simulink model "controller_test_2006"  (Simulink 6.4)
settings: Solver=ode45  StartTime=0.0  StopTime=10.0  RelTol=1e-3
values from neighbouring files (symbols this model uses):
  fundamental_sample_time = 0.01    [param_list.m]
  motor_stopped_value = DA_max / 2    [param_list.m]
libraries: simulink x1
settings Model: LastModifiedBy=Developer

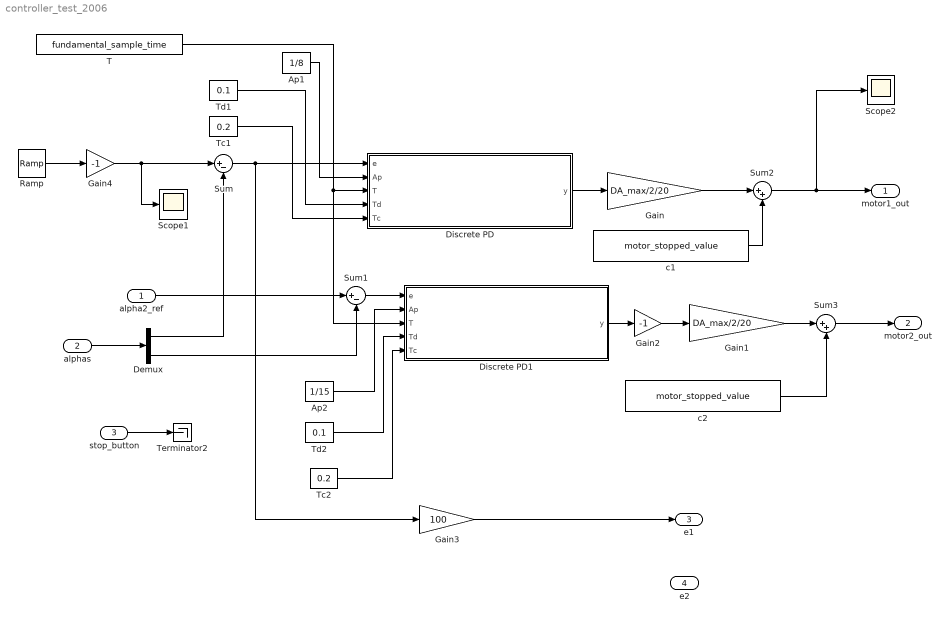
== system controller_test_2006 ==
  alpha2_ref : Inport
  alphas : Inport  Port=2
  stop_button : Inport  Port=3
  Ap1 : Constant  Value=1/8  OutDataType=sfix(16)  ConRadixGroup=Use specified scaling  OutScaling=2^0  SampleTime=inf  FramePeriod=inf
  Ap2 : Constant  Value=1/15  OutDataType=sfix(16)  ConRadixGroup=Use specified scaling  OutScaling=2^0  SampleTime=inf  FramePeriod=inf
  Demux : Demux  Outputs=2
  Discrete PD : Subsystem
  Discrete PD1 : Subsystem
  Gain : Gain  Gain=DA_max/2/20
  Gain1 : Gain  Gain=DA_max/2/20
  Gain2 : Gain  Gain=-1
  Gain3 : Gain  Gain=100
  Gain4 : Gain  Gain=-1
  Ramp : simulink/Sources/Ramp  SystemSampleTime=-1  slope=1  start=0  X0=0
  Scope1 : Scope
  Scope2 : Scope
  Sum : Sum  Inputs=|+-
  Sum1 : Sum  Inputs=|+-
  Sum2 : Sum  Inputs=|++
  Sum3 : Sum  Inputs=|++
  T : Constant  Value=fundamental_sample_time  OutDataType=sfix(16)  ConRadixGroup=Use specified scaling  OutScaling=2^0  SampleTime=inf  FramePeriod=inf
  Tc1 : Constant  Value=0.2  OutDataType=sfix(16)  ConRadixGroup=Use specified scaling  OutScaling=2^0  SampleTime=inf  FramePeriod=inf
  Tc2 : Constant  Value=0.2  OutDataType=sfix(16)  ConRadixGroup=Use specified scaling  OutScaling=2^0  SampleTime=inf  FramePeriod=inf
  Td1 : Constant  Value=0.1  OutDataType=sfix(16)  ConRadixGroup=Use specified scaling  OutScaling=2^0  SampleTime=inf  FramePeriod=inf
  Td2 : Constant  Value=0.1  OutDataType=sfix(16)  ConRadixGroup=Use specified scaling  OutScaling=2^0  SampleTime=inf  FramePeriod=inf
  Terminator2 : Terminator
  c1 : Constant  Value=motor_stopped_value  OutDataType=sfix(16)  ConRadixGroup=Use specified scaling  OutScaling=2^0  SampleTime=inf  FramePeriod=inf
  c2 : Constant  Value=motor_stopped_value  OutDataType=sfix(16)  ConRadixGroup=Use specified scaling  OutScaling=2^0  SampleTime=inf  FramePeriod=inf
  motor1_out : Outport
  motor2_out : Outport  Port=2
  e1 : Outport  Port=3
  e2 : Outport  Port=4
  wires:
  stop_button/1 -> Terminator2/1
  alphas/1 -> Demux/1
  Ramp/1 -> Gain4/1
  Sum/1 -> Discrete PD/1(e), Gain3/1
  Ap1/1 -> Discrete PD/2(Ap)
  T/1 -> Discrete PD/3(T), Discrete PD1/3(T)
  Td1/1 -> Discrete PD/4(Td)
  Tc1/1 -> Discrete PD/5(Tc)
  Demux/1 -> Sum/2
  Sum1/1 -> Discrete PD1/1(e)
  alpha2_ref/1 -> Sum1/1
  Demux/2 -> Sum1/2
  Ap2/1 -> Discrete PD1/2(Ap)
  Td2/1 -> Discrete PD1/4(Td)
  Tc2/1 -> Discrete PD1/5(Tc)
  Discrete PD1/1(y) -> Gain2/1
  Gain2/1 -> Gain1/1
  Gain3/1 -> e1/1
  Discrete PD/1(y) -> Gain/1
  c1/1 -> Sum2/2
  Gain/1 -> Sum2/1
  Sum2/1 -> motor1_out/1, Scope2/1
  Gain4/1 -> Sum/1, Scope1/1
  c2/1 -> Sum3/2
  Gain1/1 -> Sum3/1
  Sum3/1 -> motor2_out/1

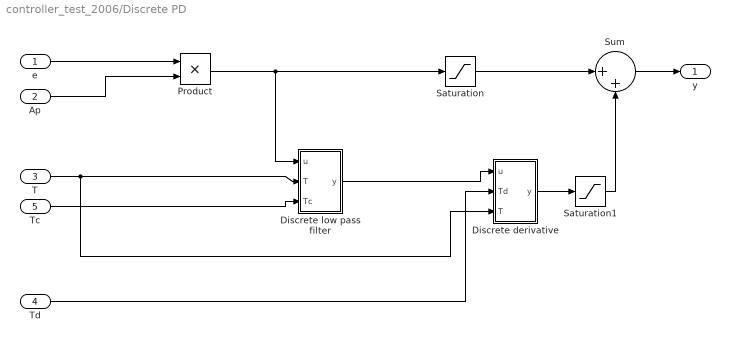
== system controller_test_2006/Discrete PD ==
  e : Inport  OutDataType=fixdt(1,16,0)  OutScaling=[]
  Ap : Inport  Port=2  OutDataType=fixdt(1,16,0)  OutScaling=[]
  T : Inport  Port=3  OutDataType=fixdt(1,16,0)  OutScaling=[]
  Td : Inport  Port=4  OutDataType=fixdt(1,16,0)  OutScaling=[]
  Tc : Inport  Port=5  OutDataType=fixdt(1,16,0)  OutScaling=[]
  Discrete derivative : Subsystem
  Discrete low pass filter : Subsystem
  Product : Product  OutDataType=fixdt(1,16,0)  OutScaling=[]  RndMeth=Zero
  Saturation : Saturate
  Saturation1 : Saturate
  Sum : Sum  Inputs=|++  OutDataType=fixdt(1,16,0)  OutScaling=[]
  y : Outport  OutDataType=fixdt(1,16,0)  OutScaling=[]
  wires:
  Product/1 -> Discrete low pass filter/1(u), Saturation/1
  e/1 -> Product/1
  Sum/1 -> y/1
  Ap/1 -> Product/2
  T/1 -> Discrete low pass filter/2(T), Discrete derivative/3(T)
  Tc/1 -> Discrete low pass filter/3(Tc)
  Td/1 -> Discrete derivative/2(Td)
  Discrete derivative/1(y) -> Saturation1/1
  Discrete low pass filter/1(y) -> Discrete derivative/1(u)
  Saturation/1 -> Sum/1
  Saturation1/1 -> Sum/2

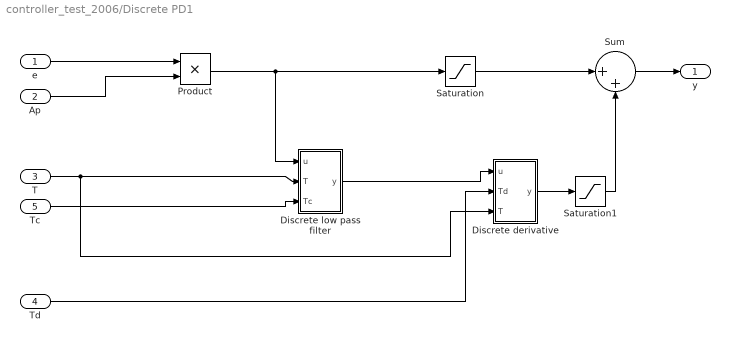
== system controller_test_2006/Discrete PD1 ==
  e : Inport  OutDataType=fixdt(1,16,0)  OutScaling=[]
  Ap : Inport  Port=2  OutDataType=fixdt(1,16,0)  OutScaling=[]
  T : Inport  Port=3  OutDataType=fixdt(1,16,0)  OutScaling=[]
  Td : Inport  Port=4  OutDataType=fixdt(1,16,0)  OutScaling=[]
  Tc : Inport  Port=5  OutDataType=fixdt(1,16,0)  OutScaling=[]
  Discrete derivative : Subsystem
  Discrete low pass filter : Subsystem
  Product : Product  OutDataType=fixdt(1,16,0)  OutScaling=[]  RndMeth=Zero
  Saturation : Saturate
  Saturation1 : Saturate
  Sum : Sum  Inputs=|++  OutDataType=fixdt(1,16,0)  OutScaling=[]
  y : Outport  OutDataType=fixdt(1,16,0)  OutScaling=[]
  wires:
  Product/1 -> Discrete low pass filter/1(u), Saturation/1
  e/1 -> Product/1
  Sum/1 -> y/1
  Ap/1 -> Product/2
  T/1 -> Discrete low pass filter/2(T), Discrete derivative/3(T)
  Tc/1 -> Discrete low pass filter/3(Tc)
  Td/1 -> Discrete derivative/2(Td)
  Discrete derivative/1(y) -> Saturation1/1
  Discrete low pass filter/1(y) -> Discrete derivative/1(u)
  Saturation/1 -> Sum/1
  Saturation1/1 -> Sum/2

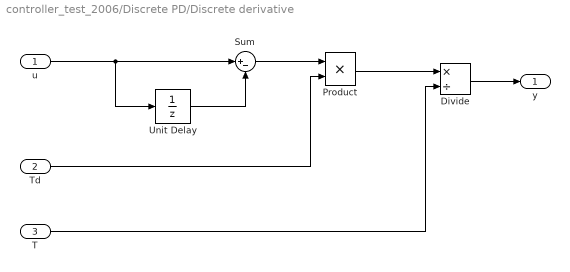
== system controller_test_2006/Discrete PD/Discrete derivative ==
  u : Inport  OutDataType=fixdt(1,16,0)  OutScaling=[]
  Td : Inport  Port=2  OutDataType=fixdt(1,16,0)  OutScaling=[]
  T : Inport  Port=3  OutDataType=fixdt(1,16,0)  OutScaling=[]
  Divide : Product  Inputs=*/  OutScaling=2^-10
  Product : Product  RndMeth=Zero
  Sum : Sum  Inputs=|+-
  Unit Delay : UnitDelay  SampleTime=-1
  y : Outport  OutDataType=fixdt(1,16,0)  OutScaling=[]
  wires:
  u/1 -> Unit Delay/1, Sum/1
  Unit Delay/1 -> Sum/2
  Sum/1 -> Product/1
  Td/1 -> Product/2
  Product/1 -> Divide/1
  T/1 -> Divide/2
  Divide/1 -> y/1

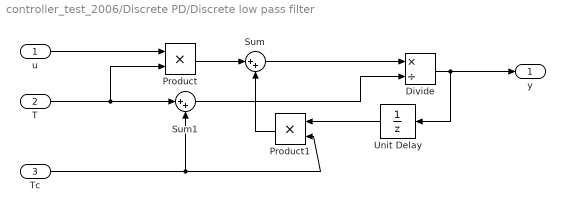
== system controller_test_2006/Discrete PD/Discrete low pass filter ==
  u : Inport  OutDataType=fixdt(1,16,0)  OutScaling=[]
  T : Inport  Port=2  OutDataType=fixdt(1,16,0)  OutScaling=[]
  Tc : Inport  Port=3  OutDataType=fixdt(1,16,0)  OutScaling=[]
  Divide : Product  Inputs=*/  OutScaling=2^-10
  Product : Product  RndMeth=Zero
  Product1 : Product  Orientation=left  RndMeth=Zero
  Sum : Sum  Inputs=|++
  Sum1 : Sum  Inputs=|++
  Unit Delay : UnitDelay  Orientation=left  SampleTime=-1
  y : Outport  OutDataType=fixdt(1,16,0)  OutScaling=[]
  wires:
  u/1 -> Product/1
  T/1 -> Product/2, Sum1/1
  Unit Delay/1 -> Product1/1
  Tc/1 -> Product1/2, Sum1/2
  Product/1 -> Sum/1
  Product1/1 -> Sum/2
  Sum/1 -> Divide/1
  Sum1/1 -> Divide/2
  Divide/1 -> Unit Delay/1, y/1

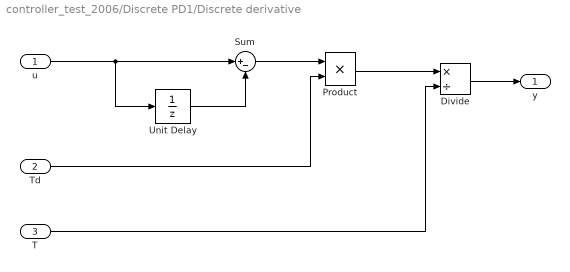
== system controller_test_2006/Discrete PD1/Discrete derivative ==
  u : Inport  OutDataType=fixdt(1,16,0)  OutScaling=[]
  Td : Inport  Port=2  OutDataType=fixdt(1,16,0)  OutScaling=[]
  T : Inport  Port=3  OutDataType=fixdt(1,16,0)  OutScaling=[]
  Divide : Product  Inputs=*/  OutScaling=2^-10
  Product : Product  RndMeth=Zero
  Sum : Sum  Inputs=|+-
  Unit Delay : UnitDelay  SampleTime=-1
  y : Outport  OutDataType=fixdt(1,16,0)  OutScaling=[]
  wires:
  u/1 -> Unit Delay/1, Sum/1
  Unit Delay/1 -> Sum/2
  Sum/1 -> Product/1
  Td/1 -> Product/2
  Product/1 -> Divide/1
  T/1 -> Divide/2
  Divide/1 -> y/1

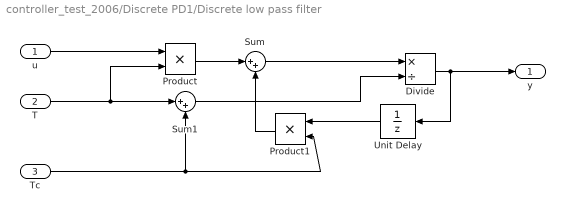
== system controller_test_2006/Discrete PD1/Discrete low pass filter ==
  u : Inport  OutDataType=fixdt(1,16,0)  OutScaling=[]
  T : Inport  Port=2  OutDataType=fixdt(1,16,0)  OutScaling=[]
  Tc : Inport  Port=3  OutDataType=fixdt(1,16,0)  OutScaling=[]
  Divide : Product  Inputs=*/  OutScaling=2^-10
  Product : Product  RndMeth=Zero
  Product1 : Product  Orientation=left  RndMeth=Zero
  Sum : Sum  Inputs=|++
  Sum1 : Sum  Inputs=|++
  Unit Delay : UnitDelay  Orientation=left  SampleTime=-1
  y : Outport  OutDataType=fixdt(1,16,0)  OutScaling=[]
  wires:
  u/1 -> Product/1
  T/1 -> Product/2, Sum1/1
  Unit Delay/1 -> Product1/1
  Tc/1 -> Product1/2, Sum1/2
  Product/1 -> Sum/1
  Product1/1 -> Sum/2
  Sum/1 -> Divide/1
  Sum1/1 -> Divide/2
  Divide/1 -> Unit Delay/1, y/1
